simulink model "sgMdl_EtherCAT_Emulator_TwinCAT"  (R2024b)
settings: Solver=FixedStepAuto  StartTime=0.0  StopTime=inf  RelTol=1e-3
libraries: speedgoatlib_ecatsim x9, simulink x2
Description:
  | EtherCAT - Emulator with TwinCAT
settings Model: ModifiedByFormat=Speedgoat  Creator=Speedgoat  LastModifiedBy=Speedgoat
settings SolverCC: ConcurrentTasks=on  PositivePriorityOrder=on
settings OptimizationCC: BlockReduction=off  OptimizeBlockIOStorage=off
settings DebuggingCC: TasksWithSamePriorityMsg=none
settings HardwareCC: ProdBitPerLong=64  ProdLongLongMode=on  ProdHWDeviceType=Intel->x86-64 (Linux 64)
settings RTWCC: Description=Speedgoat Real-Time Target Machine  SystemTargetFile=speedgoat.tlc  TemplateMakefile=slrealtime_default_tmf  Toolchain=Simulink Real-Time Toolchain  BuildConfiguration=Faster Runs  TargetLang=C++
settings SimulinkRealTimeTargetCC: SubcomponentCodeInterfacePackaging=Reusable function  MATLABClassNameForMDSCustomization=Simulink.SoftwareTarget.GRTCustomization  InstructionSetFMA=off  LogToMDFFile=off  SLRTFileLogMaxRuns=10
settings ConfigComp: CovBoundaryAbsTol=1.0e-5

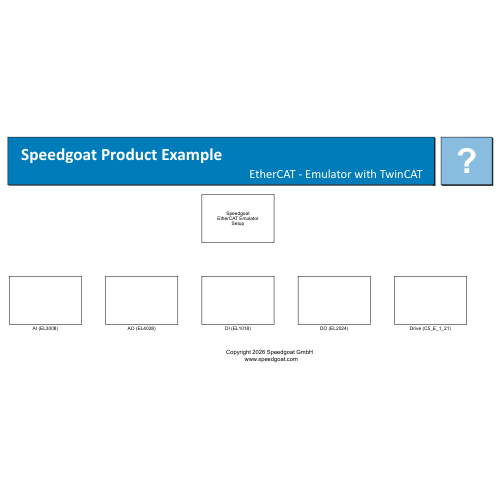
[thumbnail: Simulink's stored preview of the top-level diagram]
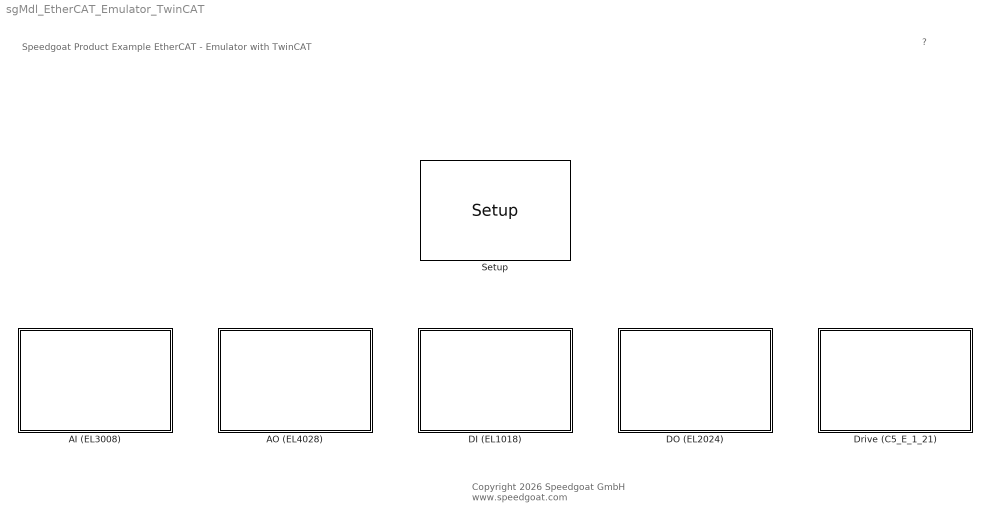
== system sgMdl_EtherCAT_Emulator_TwinCAT ==
  note: Speedgoat Product Example
      | EtherCAT - Emulator with TwinCAT
  note: ?
  note: Copyright 2026 Speedgoat GmbH
      |  www.speedgoat.com
  AI (EL3008) : Subsystem
  AO (EL4028) : Subsystem
  DI (EL1018) : Subsystem
  DO (EL2024) : Subsystem
  Drive (C5_E_1_21) : Subsystem
  "Setup " : speedgoatlib_ecatsim/Setup   parInterface=1  parFirstDevice=1001  parConfigFile=which('EtherCAT_Emulator_TwinCAT_exi.xml')

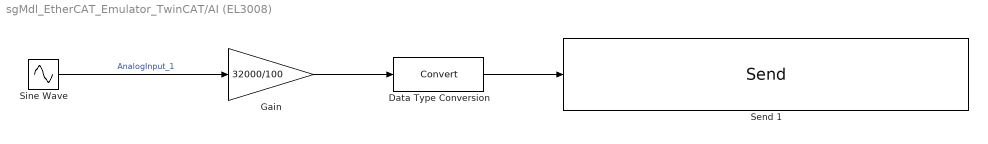
== system sgMdl_EtherCAT_Emulator_TwinCAT/AI (EL3008) ==
  Data Type Conversion : DataTypeConversion  SaturateOnIntegerOverflow=off  RndMeth=Floor
  Gain : Gain  Gain=32000/100
  Send 1 : speedgoatlib_ecatsim/Send   parInterface=1  parSlaveAddress=1002  parSignalName="{\"Term 3 (EL3008).AI Standard Channel 1.Value\"}"  parSignalDataType="{\"int16\"}"  parSignalOffset=560  parSignalWidth=1  parSampleTime=0.001
  Sine Wave : Sin  SineType=Sample based  Amplitude=30  Samples=5000  SampleTime=0.001
  wires:
  Sine Wave/1 -> Gain/1  "AnalogInput_1"
  Gain/1 -> Data Type Conversion/1
  Data Type Conversion/1 -> Send 1/1

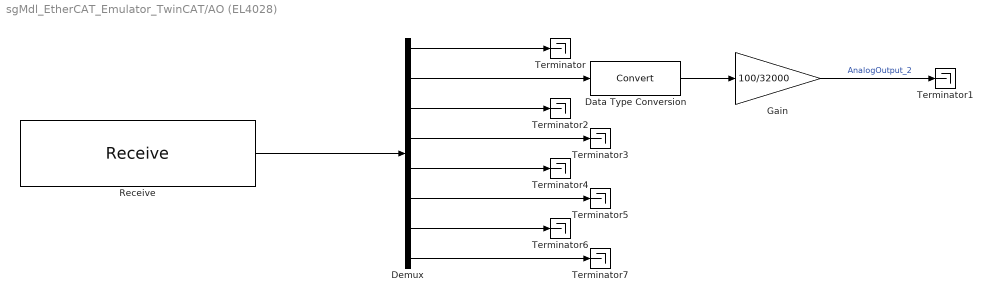
== system sgMdl_EtherCAT_Emulator_TwinCAT/AO (EL4028) ==
  Data Type Conversion : DataTypeConversion  SaturateOnIntegerOverflow=off  RndMeth=Floor
  Demux : Demux  Outputs=8
  Gain : Gain  Gain=100/32000
  "Receive " : speedgoatlib_ecatsim/Receive   parInterface=1  parSlaveAddress=1003  parSignalName={'Analog output'}  parSignalDataType="{\"int16\"}"  parSignalOffset=[312]  parSignalWidth=[8]  parSampleTime=0.001
  Terminator{,1..7} (8 alike) : Terminator
  wires:
  "Receive "/1 -> Demux/1
  Demux/1 -> Terminator/1
  Demux/2 -> Data Type Conversion/1
  Demux/3 -> Terminator2/1
  Demux/4 -> Terminator3/1
  Demux/8 -> Terminator7/1
  Demux/7 -> Terminator6/1
  Demux/6 -> Terminator5/1
  Demux/5 -> Terminator4/1
  Data Type Conversion/1 -> Gain/1
  Gain/1 -> Terminator1/1  "AnalogOutput_2"

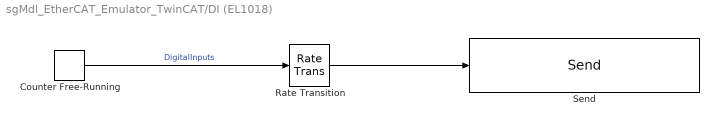
== system sgMdl_EtherCAT_Emulator_TwinCAT/DI (EL1018) ==
  Counter Free-Running : simulink/Sources/Counter Free-Running  NumBits=8  tsamp=1
  Rate Transition : RateTransition
  "Send " : speedgoatlib_ecatsim/Send   parInterface=1  parSlaveAddress=1004  parSignalName={'Input'}  parSignalDataType="{\"uint8\"}"  parSignalOffset=[800]  parSignalWidth=[1]  parSampleTime=0.001
  wires:
  Rate Transition/1 -> "Send "/1
  Counter Free-Running/1 -> Rate Transition/1  "DigitalInputs"

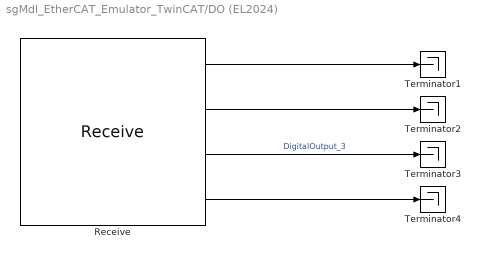
== system sgMdl_EtherCAT_Emulator_TwinCAT/DO (EL2024) ==
  "Receive " : speedgoatlib_ecatsim/Receive   parInterface=1  parSlaveAddress=1005  parSignalName={'Output_1','Output_2','Output_3','Output_4'}  parSignalDataType="{\"boolean\",\"boolean\",\"boolean\",\"boolean\"}"  parSignalOffset=[440,441,442,443]  parSignalWidth=|  parSampleTime=0.001
      | [
      | 1
      | ,
      | 1
      | ,
      | 1
      | ,
      | 1
      | ]
  Terminator{1..4} (4 alike) : Terminator
  wires:
  "Receive "/1 -> Terminator1/1
  "Receive "/2 -> Terminator2/1
  "Receive "/3 -> Terminator3/1  "DigitalOutput_3"
  "Receive "/4 -> Terminator4/1

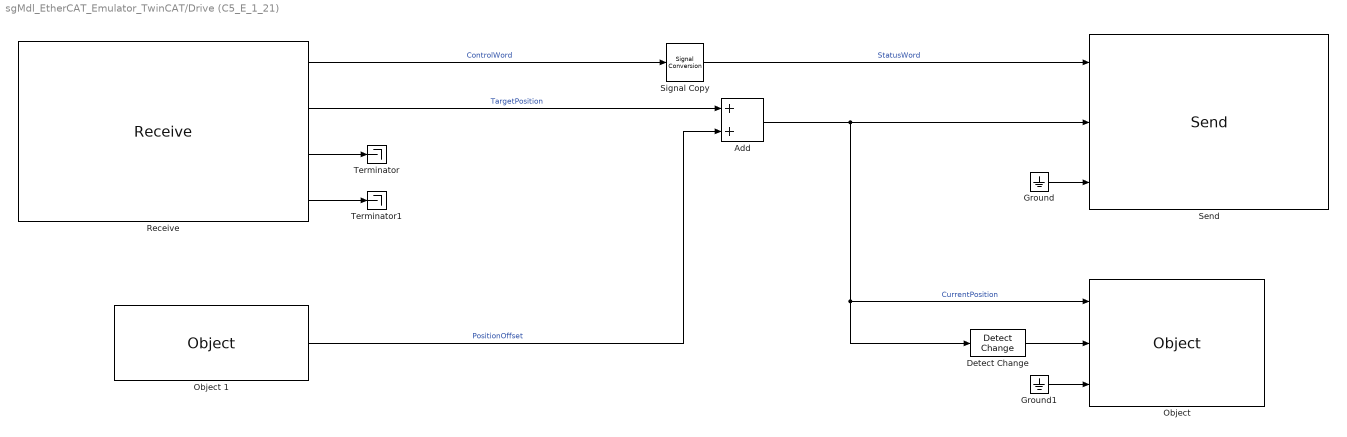
== system sgMdl_EtherCAT_Emulator_TwinCAT/Drive (C5_E_1_21) ==
  Add : Sum
  Detect Change : simulink/Logic and Bit Operations/Detect Change  vinit=0  OutDataTypeStr=boolean
  Ground : Ground
  Ground1 : Ground
  "Object " : speedgoatlib_ecatsim/Object   parInterface=1  parSlaveAddress=1006  parSdoIndex=hex2dec('6064')  parSdoSubIndex=0  parInitValue=int32(-1)  parReadOp=off  parWriteOp=on  parExtended=on  parSampleTime=0.001
  Object 1 : speedgoatlib_ecatsim/Object   parInterface=1  parSlaveAddress=1006  parSdoIndex=hex2dec('60B0')  parSdoSubIndex=0  parInitValue=int32(0)  parReadOp=on  parWriteOp=off  parExtended=off  parSampleTime=0.001
  "Receive " : speedgoatlib_ecatsim/Receive   parInterface=1  parSlaveAddress=1006  parSignalName={'Controlword','Target Position','Motor drive submode select','Modes of operation'}  parSignalDataType="{\"uint16\",\"int32\",\"uint32\",\"int8\"}"  parSignalOffset=[904,920,952,984]  parSignalWidth=|  parSampleTime=0.001
      | [
      | 1
      | ,
      | 1
      | ,
      | 1
      | ,
      | 1
      | ]
  "Send " : speedgoatlib_ecatsim/Send   parInterface=1  parSlaveAddress=1006  parSignalName={'Statusword','Position actual value','Modes of operation display'}  parSignalDataType="{\"uint16\",\"int32\",\"int8\"}"  parSignalOffset=[904,920,952]  parSignalWidth=|  parSampleTime=0.001
      | [
      | 1
      | ,
      | 1
      | ,
      | 1
      | ]
  Signal Copy : SignalConversion  OverrideOpt=off
  Terminator : Terminator
  Terminator1 : Terminator
  wires:
  "Receive "/2 -> Add/1  "TargetPosition"
  Ground/1 -> "Send "/3
  "Receive "/3 -> Terminator/1
  "Receive "/4 -> Terminator1/1
  "Receive "/1 -> Signal Copy/1  "ControlWord"
  Add/1 -> "Object "/1, Detect Change/1, "Send "/2  "CurrentPosition"
  Ground1/1 -> "Object "/3
  Detect Change/1 -> "Object "/2
  Object 1/1 -> Add/2  "PositionOffset"
  Signal Copy/1 -> "Send "/1  "StatusWord"
